simulink model "motormodel"  (Simulink 7.4)
settings: Solver=ode45  StartTime=0.0  StopTime=40.69  RelTol=1e-3
undefined symbols (not defined in the file or in its folder): Bm, Jm, Km, Rm
settings Model: Creator=HOSTRUP  LastModifiedBy=HOSTRUP

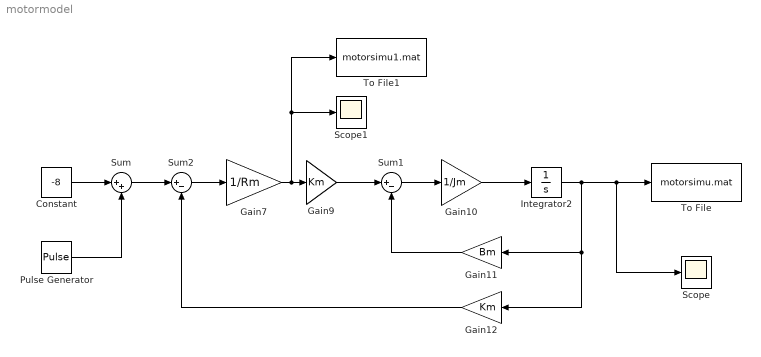
== system motormodel ==
  Constant : Constant  Value=-8  OutDataType=fixdt(1, 16)  OutScaling=2^0
  Gain10 : Gain  Gain=1/Jm  ParameterDataType=fixdt(1, 16)  ParameterScaling=2^0  OutDataType=fixdt(1, 16)  OutScaling=2^0
  Gain11 : Gain  Gain=Bm  ParameterDataType=fixdt(1, 16)  ParameterScaling=2^0  OutDataType=fixdt(1, 16)  OutScaling=2^0
  Gain12 : Gain  Gain=Km  ParameterDataType=fixdt(1, 16)  ParameterScaling=2^0  OutDataType=fixdt(1, 16)  OutScaling=2^0
  Gain7 : Gain  Gain=1/Rm  ParameterDataType=fixdt(1, 16)  ParameterScaling=2^0  OutDataType=fixdt(1, 16)  OutScaling=2^0
  Gain9 : Gain  Gain=Km  ParameterDataType=fixdt(1, 16)  ParameterScaling=2^0  OutDataType=fixdt(1, 16)  OutScaling=2^0
  Integrator2 : Integrator
  Pulse Generator : DiscretePulseGenerator  PulseType=Time based  Amplitude=16  Period=4  PulseWidth=50  PhaseDelay=0  SampleTime=1
  Scope : Scope
  Scope1 : Scope
  Sum : Sum  Inputs=|++  OutDataType=fixdt(1, 16)  OutScaling=2^0
  Sum1 : Sum  Inputs=|+-  OutDataType=fixdt(1, 16)  OutScaling=2^0
  Sum2 : Sum  Inputs=|+-  OutDataType=fixdt(1, 16)  OutScaling=2^0
  To File : ToFile  Filename=motorsimu.mat  SampleTime=0.01
  To File1 : ToFile  Filename=motorsimu1.mat  SampleTime=0.01
  wires:
  Pulse Generator/1 -> Sum/2
  Constant/1 -> Sum/1
  Gain7/1 -> Gain9/1, To File1/1, Scope1/1
  Gain10/1 -> Integrator2/1
  Sum1/1 -> Gain10/1
  Integrator2/1 -> Gain11/1, Gain12/1, To File/1, Scope/1
  Gain12/1 -> Sum2/2
  Gain11/1 -> Sum1/2
  Gain9/1 -> Sum1/1
  Sum/1 -> Sum2/1
  Sum2/1 -> Gain7/1
